simulink model "Question2_hw3"  (R2015a)
settings: Solver=ode45  StartTime=0.0  StopTime=50  RelTol=1e-3
settings Model: Creator=Burak Akyürek  LastModifiedBy=Burak Akyürek

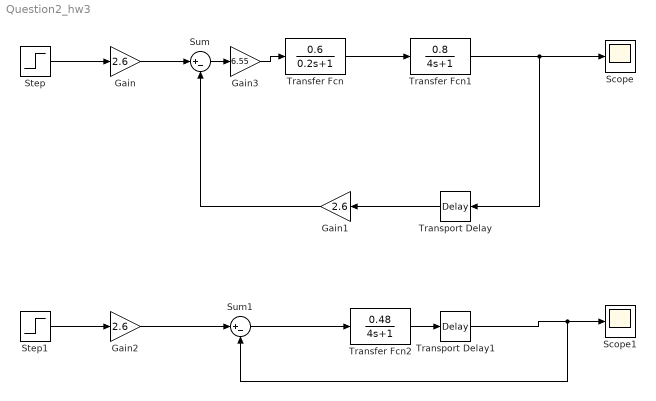
== system Question2_hw3 ==
  Gain : Gain  Gain=2.6
  Gain1 : Gain  Gain=2.6
  Gain2 : Gain  Gain=2.6
  Gain3 : Gain  Gain=6.55
  Scope : Scope
  Scope1 : Scope
  Step : Step  SampleTime=0
  Step1 : Step  SampleTime=0
  Sum : Sum  Inputs=|+-
  Sum1 : Sum  Inputs=|+-
  Transfer Fcn : TransferFcn  Numerator=[0.6]  Denominator=[0.2 1]
  Transfer Fcn1 : TransferFcn  Numerator=[0.8]  Denominator=[4 1]
  Transfer Fcn2 : TransferFcn  Numerator=[0.48]  Denominator=[4 1]
  Transport Delay : TransportDelay  DelayTime=0.725
  Transport Delay1 : TransportDelay  DelayTime=0.925
  wires:
  Step/1 -> Gain/1
  Gain/1 -> Sum/1
  Transfer Fcn/1 -> Transfer Fcn1/1
  Transfer Fcn1/1 -> Transport Delay/1, Scope/1
  Gain1/1 -> Sum/2
  Transport Delay/1 -> Gain1/1
  Step1/1 -> Gain2/1
  Transfer Fcn2/1 -> Transport Delay1/1
  Transport Delay1/1 -> Sum1/2, Scope1/1
  Gain2/1 -> Sum1/1
  Sum1/1 -> Transfer Fcn2/1
  Sum/1 -> Gain3/1
  Gain3/1 -> Transfer Fcn/1
